simulink model "lab6_zbiorniki_compare"  (R2023a)
settings: Solver=ode45  StartTime=0.0  StopTime=150.0  MaxStep=0.05  RelTol=1e-3  EnableMultiTasking=on
libraries: simulink x2
settings Model: Creator=Aneta  LastModifiedBy=bm50345
settings SolverCC: AlgebraicLoopSolver=TrustRegion
settings DataIOCC: LimitDataPoints=on  SaveFormat=Array  ReturnWorkspaceOutputs=off
settings OptimizationCC: ExpressionDepthLimit=2147483647  LifeSpan=inf
settings DebuggingCC: UnderspecifiedInitializationDetection=Classic  MergeDetectMultiDrivingBlocksExec=none  SolverPrmCheckMsg=warning  UnconnectedInputMsg=warning  UnconnectedOutputMsg=warning  UnconnectedLineMsg=warning  StateNameClashWarn=warning  SFUnexpectedBacktrackingDiag=warning  SFNoUnconditionalDefaultTransitionDiag=warning  SFExecutionAtInitializationDiag=none  ArithmeticOperatorsInVariantConditions=warning
settings HardwareCC: ProdBitPerPointer=32  ProdBitPerSizeT=32  ProdBitPerPtrDiffT=32  ProdLargestAtomicFloat=None  ProdIntDivRoundTo=Undefined  ProdEndianess=Unspecified  ProdWordSize=32  ProdHWDeviceType=32-bit Generic
settings ModelReferenceCC: EnableRefExpFcnMdlSchedulingChecks=on  PropagateSignalLabelsOutOfModel=off
settings SFSimCC: SimUseLocalCustomCode=off  CustomCodeUndefinedFunction=UseInterfaceOnly
settings RTWCC: RTWUseLocalCustomCode=off  DLArmComputeVersion=19.05
settings CodeAppCC: StateflowObjectComments=on
settings GRTTargetCC: TargetLangStandard=C89/C90 (ANSI)
settings ConfigComp: CovMetricSettings=dw  CovSaveCumulativeToWorkspaceVar=on  CovSaveSingleToWorkspaceVar=on  CovExternalEMLEnable=off

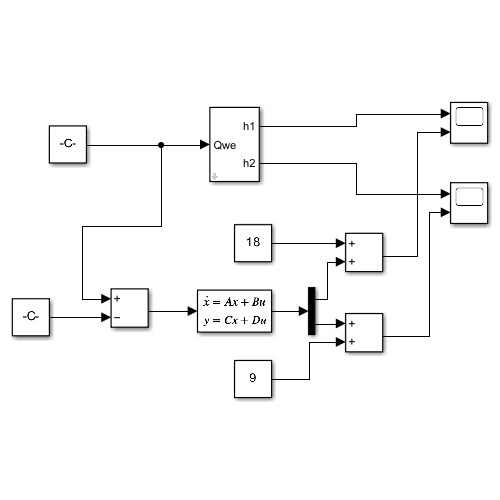
[thumbnail: Simulink's stored preview of the top-level diagram]
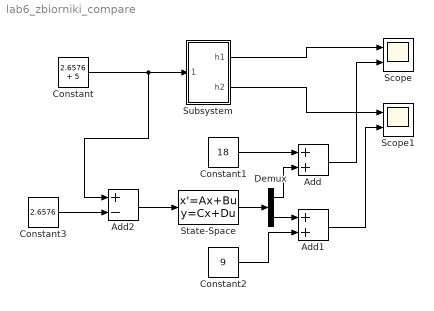
== system lab6_zbiorniki_compare ==
  Add : Sum
  Add1 : Sum
  Add2 : Sum  Inputs=+-
  Constant : Constant  Value=2.6576 + 5
  Constant1 : Constant  Value=18
  Constant2 : Constant  Value=9
  Constant3 : Constant  Value=2.6576
  Demux : Demux  Outputs=2
  Scope : Scope  NumInputPorts=2
  Scope1 : Scope  NumInputPorts=2
  State-Space : StateSpace  A=[-0.147648230610174,0.147648230603981;0.073824115305087,-0.147648230603981]  B=[1;0]  C=[1,0;0,1]  D=[0;0]  InitialCondition=[-14,-7]
  Subsystem : Subsystem  mask{h1=4, h2=2, S1=1, S2=2, Swy1=0.2, Swy2=0.2, fi1=1, fi2=1, g=9.81, Qwe=2}
  wires:
  Constant/1 -> Add2/1, Subsystem/1(Qwe)
  Subsystem/1(h1) -> Scope/1
  Subsystem/2(h2) -> Scope1/1
  Add/1 -> Scope/2
  Constant1/1 -> Add/1
  State-Space/1 -> Demux/1
  Demux/1 -> Add/2
  Demux/2 -> Add1/1
  Constant2/1 -> Add1/2
  Add1/1 -> Scope1/2
  Add2/1 -> State-Space/1
  Constant3/1 -> Add2/2

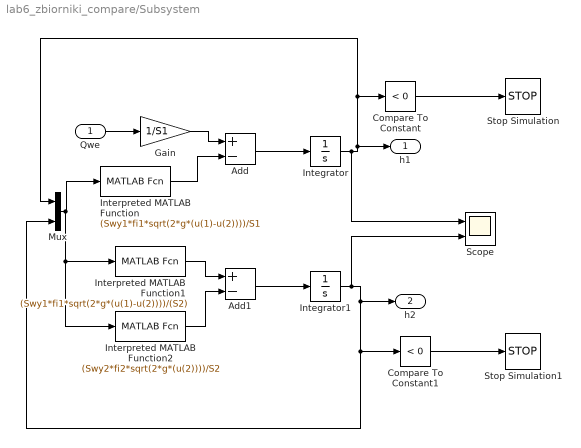
== system lab6_zbiorniki_compare/Subsystem ==
  Qwe : Inport
  Add : Sum  Inputs=+-
  Add1 : Sum  Inputs=+-
  Compare To Constant : simulink/Logic and Bit Operations/Compare To Constant  relop=<  const=0  OutDataTypeStr=boolean
  Compare To Constant1 : simulink/Logic and Bit Operations/Compare To Constant  relop=<  const=0  OutDataTypeStr=boolean
  Gain : Gain  Gain=1/S1
  Integrator : Integrator  InitialCondition=h1
  Integrator1 : Integrator  InitialCondition=h2
  Interpreted MATLAB Function : MATLABFcn  MATLABFcn=(Swy1*fi1*sqrt(2*g*(u(1)-u(2))))/S1
  Interpreted MATLAB Function1 : MATLABFcn  MATLABFcn=(Swy1*fi1*sqrt(2*g*(u(1)-u(2))))/(S2)
  Interpreted MATLAB Function2 : MATLABFcn  MATLABFcn=(Swy2*fi2*sqrt(2*g*(u(2))))/S2
  Mux : Mux  Inputs=2
  Scope : Scope  NumInputPorts=2
  Stop Simulation : Stop
  Stop Simulation1 : Stop
  h1 : Outport
  h2 : Outport  Port=2
  wires:
  Integrator/1 -> Scope/1, h1/1, Compare To Constant/1, Mux/1
  Add1/1 -> Integrator1/1
  Add/1 -> Integrator/1
  Interpreted MATLAB Function/1 -> Add/2
  Mux/1 -> Interpreted MATLAB Function2/1, Interpreted MATLAB Function1/1, Interpreted MATLAB Function/1
  Interpreted MATLAB Function2/1 -> Add1/2
  Interpreted MATLAB Function1/1 -> Add1/1
  Compare To Constant/1 -> Stop Simulation/1
  Integrator1/1 -> Scope/2, h2/1, Compare To Constant1/1, Mux/2
  Compare To Constant1/1 -> Stop Simulation1/1
  Gain/1 -> Add/1
  Qwe/1 -> Gain/1
